simulink model "soc_WLAN_fpga"  (R2024b)
settings: Solver=FixedStepDiscrete  StartTime=0.0  StopTime=stopTime  RelTol=1e-3
PreLoadFcn:
  | addpath(fullfile(matlabroot,'toolbox','whdl','whdlexamples','whdlexamples'));
InitFcn:
  | addpath(fullfile(matlabroot,'toolbox','whdl','whdlexamples','whdlexamples'));
model workspace (MAT data in the model file):
  socvcb : containers.Map (value not decoded)
undefined symbols (not defined in the file): Add, bitRatePerOfdmSym, chanBW, coe, cpLen, dataUpsampleFactor, DelayValMaxNsdMinusLastPilotSc, DescramblerInitialSeed, designMultirateFIR, fftLen, filterLatency, filterUpsampleFactor, Fs, Hd, HT_MFMCS0, HT_MFMCS1, HT_MFMCS2, HT_MFMCS3, HT_MFMCS4, HT_MFMCS5, HT_MFMCS6, HT_MFMCS7, HTUnUsedScInd, inputSamplingRate, interp_coeff, maxPilotRefCounterVale, maxPilotsRef, maxPilotsRefNonHT, Ncol_HT, Ncol_NonHT, noDataSubCarriers, Non_HTMCS0, Non_HTMCS1, Non_HTMCS2, Non_HTMCS3, Non_HTMCS4, Non_HTMCS5, Non_HTMCS6, Non_HTMCS7, Nrow_HT, Nrow_NonHT, numDSC_HT, numDSC_HT_vhtSigB, numDSC_NonHT, numDscHT, numDscNonHT, numOfBitsPerOFDMSym, numOfDataBitsPerOFDMSym, numPilots, numScHT, numSCS_HT, numSCS_NonHT, pnSeq, QAM, rxDownsampleFactor, secondPIdx_HT, secondPIdx_NonHT, Shift, VHTMCS0, VHTMCS1 ... (+7)
libraries: hdlsllib x267, simulink x210, dspsigops x22, whdlutilities x10, whdlmod x9, dsphdlfiltering2 x5, dsphdlmathfun2 x4, whdledac x3, hwlogicconnlib x2, commhdlcrc x2, dsphdlsigops2 x2
(part 13 of 14)

== system soc_WLAN_fpga/WLAN/WLAN HDL/WLAN_Tx_Rx/WLAN_Rx/WLANHDLReceiver/DataRecovery/Deinterleaver/DeInterleaver_NonHT/Stage 2 64QAM/Read Logic/Generate Read Address/Read Address of Deinterleaver/Generate Read Address ==
  note: Compute read address
  blockLen : Inport
  enable : Inport  Port=2
  reset : Inport  Port=3
  Add : Sum
  Add1 : Sum  OutDataTypeStr=fixdt(0,nextpow2(maxBlkSize),0)
  Constant : Constant  OutDataTypeStr=fixdt(0,1,0)  SampleTime=-1
  Constant1 : Constant  Value=nColumns-2  OutDataTypeStr=Inherit: Inherit via back propagation  SampleTime=-1
  Constant2 : Constant  Value=nColumns  OutDataTypeStr=fixdt(0,nextpow2(nColumns+1),0)  SampleTime=-1
  Constant4 : Constant  Value=nColumns  OutDataTypeStr=Inherit: Inherit via back propagation  SampleTime=-1
  Delay{,4..6,10..12,14..16} (10 alike) : Delay  DelayLength=1
  Delay{1..3,13} (4 alike) : Delay
  Divide : Product  Inputs=*/  OutDataTypeStr=fixdt(0,nextpow2(maxNRows+1),0)  RndMeth=Zero  SaturateOnIntegerOverflow=on
  From : From
  Goto : Goto
  HDL Counter2 : hdlsllib/Sources/HDL Counter  CountType=Count limited  CountInit=0  CountStep=1  CountMax=maxBlkSize  CountFromType=Initial value  CountFrom=0  CountResetPort=on  CountLoadPort=off  CountEnbPort=on  CountDirPort=off  CountHitOutputPort=off  CountDataType=Unsigned  CountWordLen=nextpow2(maxBlkSize+1)  CountFracLen=0  CountSampTime=1
  Logical Operator : Logic  Operator=OR  IconShape=distinctive  AllPortsSameDT=off  OutDataTypeStr=boolean
  Logical Operator1 : Logic  IconShape=distinctive  AllPortsSameDT=off  OutDataTypeStr=boolean
  Product : Product  OutDataTypeStr=fixdt(0,nextpow2(maxBlkSize),0)
  Relational Operator : RelationalOperator  Operator===  OutDataTypeStr=boolean  InputSameDT=off
  Relational Operator1 : RelationalOperator  OutDataTypeStr=boolean  InputSameDT=off
  Switch : Switch  Criteria=u2 ~= 0  SaturateOnIntegerOverflow=off  InputSameDT=off
  colCounter : hdlsllib/Sources/HDL Counter  CountType=Count limited  CountInit=0  CountStep=1  CountMax=maxNRows -1  CountFromType=Initial value  CountFrom=0  CountResetPort=on  CountLoadPort=off  CountEnbPort=on  CountDirPort=off  CountHitOutputPort=off  CountDataType=Unsigned  CountWordLen=nextpow2(maxNRows)  CountFracLen=0  CountSampTime=1
  rowCounter : hdlsllib/Sources/HDL Counter  CountType=Count limited  CountInit=0  CountStep=1  CountMax=nColumns -1  CountFromType=Initial value  CountFrom=0  CountResetPort=on  CountLoadPort=off  CountEnbPort=on  CountDirPort=off  CountHitOutputPort=off  CountDataType=Unsigned  CountWordLen=nextpow2(nColumns+1)  CountFracLen=0  CountSampTime=1
  blockDataCount : Outport
  currentAddr : Outport  Port=2
  wires:
  Relational Operator1/1 -> Logical Operator1/1
  HDL Counter2/1 -> Goto/1, Relational Operator1/2
  reset/1 -> Delay15/1, HDL Counter2/1
  Logical Operator/1 -> rowCounter/1
  Delay/1 -> Logical Operator/1, colCounter/2
  Relational Operator/1 -> Delay/1
  Constant/1 -> Add/2
  blockLen/1 -> Relational Operator1/1, Add/1
  enable/1 -> Logical Operator1/2, HDL Counter2/2
  rowCounter/1 -> Delay1/1, Relational Operator/2  "rowIndex"
  colCounter/1 -> Delay2/1  "colIndex"
  Add1/1 -> Delay6/1
  Product/1 -> Delay5/1
  Delay2/1 -> Delay4/1
  Delay4/1 -> Add1/2
  Delay5/1 -> Add1/1
  Delay15/1 -> colCounter/1, Logical Operator/2
  Delay16/1 -> Switch/2, rowCounter/2
  Delay13/1 -> Delay14/1
  Delay14/1 -> Delay11/1
  Delay12/1 -> Delay13/1
  Delay6/1 -> currentAddr/1
  Delay11/1 -> blockDataCount/1
  Add/1 -> Delay10/1
  From/1 -> Delay12/1
  Logical Operator1/1 -> Delay16/1
  Divide/1 -> Delay3/1
  Delay10/1 -> Divide/1
  Constant2/1 -> Divide/2
  Switch/1 -> Relational Operator/1
  Constant1/1 -> Switch/1
  Constant4/1 -> Switch/3
  Delay1/1 -> Product/2
  Delay3/1 -> Product/1

== system soc_WLAN_fpga/WLAN/WLAN HDL/WLAN_Tx_Rx/WLAN_Rx/WLANHDLReceiver/DataRecovery/Deinterleaver/DeInterleaver_NonHT/Stage 2 64QAM/Read Logic/Generate Read Address/Read Address of Interleaver/Generate Read Address ==
  note: Compute read address
  blockLen : Inport
  enable : Inport  Port=2
  reset : Inport  Port=3
  Add : Sum
  Add1 : Sum  Inputs=+-  OutDataTypeStr=Inherit: Inherit via back propagation
  Add2 : Sum  OutDataTypeStr=fixdt(0,nextpow2(maxBlkSize),0)
  Constant : Constant  OutDataTypeStr=fixdt(0,1,0)  SampleTime=-1
  Constant1 : Constant  Value=2  OutDataTypeStr=fixdt(0,2,0)  SampleTime=-1
  Constant2 : Constant  Value=nColumns  OutDataTypeStr=fixdt(0,nextpow2(nColumns+1),0)  SampleTime=-1
  Constant3 : Constant  Value=nColumns  OutDataTypeStr=fixdt(0,nextpow2(nColumns+1),0)  SampleTime=-1
  Constant4 : Constant  Value=maxNRows  OutDataTypeStr=Inherit: Inherit via back propagation  SampleTime=-1
  Delay{,1..16} (17 alike) : Delay  DelayLength=1
  Divide : Product  Inputs=*/  OutDataTypeStr=fixdt(0,nextpow2(maxNRows+1),0)  RndMeth=Zero  SaturateOnIntegerOverflow=on
  From : From
  Goto : Goto
  HDL Counter2 : hdlsllib/Sources/HDL Counter  CountType=Count limited  CountInit=0  CountStep=1  CountMax=maxBlkSize  CountFromType=Initial value  CountFrom=0  CountResetPort=on  CountLoadPort=off  CountEnbPort=on  CountDirPort=off  CountHitOutputPort=off  CountDataType=Unsigned  CountWordLen=nextpow2(maxBlkSize+1)  CountFracLen=0  CountSampTime=1
  Logical Operator : Logic  Operator=OR  IconShape=distinctive  AllPortsSameDT=off  OutDataTypeStr=boolean
  Logical Operator1 : Logic  IconShape=distinctive  AllPortsSameDT=off  OutDataTypeStr=boolean
  Product : Product  OutDataTypeStr=fixdt(0,nextpow2(maxBlkSize),0)
  Relational Operator : RelationalOperator  Operator===  OutDataTypeStr=boolean  InputSameDT=off
  Relational Operator1 : RelationalOperator  OutDataTypeStr=boolean  InputSameDT=off
  Switch : Switch  Criteria=u2 ~= 0  SaturateOnIntegerOverflow=off  InputSameDT=off
  colCounter : hdlsllib/Sources/HDL Counter  CountType=Count limited  CountInit=0  CountStep=1  CountMax=nColumns -1  CountFromType=Initial value  CountFrom=0  CountResetPort=on  CountLoadPort=off  CountEnbPort=on  CountDirPort=off  CountHitOutputPort=off  CountDataType=Unsigned  CountWordLen=nextpow2(nColumns)  CountFracLen=0  CountSampTime=1
  rowCounter : hdlsllib/Sources/HDL Counter  CountType=Count limited  CountInit=0  CountStep=1  CountMax=maxNRows -1  CountFromType=Initial value  CountFrom=0  CountResetPort=on  CountLoadPort=off  CountEnbPort=on  CountDirPort=off  CountHitOutputPort=off  CountDataType=Unsigned  CountWordLen=nextpow2(maxNRows+1)  CountFracLen=0  CountSampTime=1
  blockDataCount : Outport
  currentAddr : Outport  Port=2
  wires:
  Constant3/1 -> Product/2
  Delay9/1 -> Delay13/1
  Delay8/1 -> rowCounter/2, Switch/2
  Delay7/1 -> Logical Operator/2, colCounter/1
  Delay3/1 -> Add1/1
  Delay1/1 -> Product/1
  Add1/1 -> Switch/1
  Constant1/1 -> Add1/2
  Divide/1 -> Delay3/1
  Constant4/1 -> Switch/3
  Switch/1 -> Relational Operator/1
  Constant2/1 -> Divide/2
  Delay10/1 -> Divide/1
  Logical Operator1/1 -> Delay16/1
  From/1 -> Delay12/1
  Add/1 -> Delay10/1
  Delay11/1 -> blockDataCount/1
  Delay6/1 -> currentAddr/1
  Delay12/1 -> Delay9/1
  Delay14/1 -> Delay11/1
  Delay13/1 -> Delay14/1
  Delay16/1 -> Delay8/1
  Delay15/1 -> Delay7/1
  Delay5/1 -> Add2/1
  Delay4/1 -> Add2/2
  Delay2/1 -> Delay4/1
  Product/1 -> Delay5/1
  Add2/1 -> Delay6/1
  colCounter/1 -> Delay2/1  "colIndex"
  rowCounter/1 -> Delay1/1, Relational Operator/2  "rowIndex"
  enable/1 -> HDL Counter2/2, Logical Operator1/2
  blockLen/1 -> Add/1, Relational Operator1/1
  Constant/1 -> Add/2
  Relational Operator/1 -> Delay/1
  Delay/1 -> colCounter/2, Logical Operator/1
  Logical Operator/1 -> rowCounter/1
  reset/1 -> HDL Counter2/1, Delay15/1
  HDL Counter2/1 -> Relational Operator1/2, Goto/1
  Relational Operator1/1 -> Logical Operator1/1

== system soc_WLAN_fpga/WLAN/WLAN HDL/WLAN_Tx_Rx/WLAN_Rx/WLANHDLReceiver/DataRecovery/Deinterleaver/DeInterleaver_NonHT/Stage 2 BPSK/Read Logic/Generate Read Address/Read Address of Deinterleaver/Generate Read Address ==
  note: Compute read address
  blockLen : Inport
  enable : Inport  Port=2
  reset : Inport  Port=3
  Add : Sum
  Add1 : Sum  OutDataTypeStr=fixdt(0,nextpow2(maxBlkSize),0)
  Constant : Constant  OutDataTypeStr=fixdt(0,1,0)  SampleTime=-1
  Constant1 : Constant  Value=nColumns-2  OutDataTypeStr=Inherit: Inherit via back propagation  SampleTime=-1
  Constant2 : Constant  Value=nColumns  OutDataTypeStr=fixdt(0,nextpow2(nColumns+1),0)  SampleTime=-1
  Constant4 : Constant  Value=nColumns  OutDataTypeStr=Inherit: Inherit via back propagation  SampleTime=-1
  Delay{,4..6,10..12,14..16} (10 alike) : Delay  DelayLength=1
  Delay{1..3,13} (4 alike) : Delay
  Divide : Product  Inputs=*/  OutDataTypeStr=fixdt(0,nextpow2(maxNRows+1),0)  RndMeth=Zero  SaturateOnIntegerOverflow=on
  From : From
  Goto : Goto
  HDL Counter2 : hdlsllib/Sources/HDL Counter  CountType=Count limited  CountInit=0  CountStep=1  CountMax=maxBlkSize  CountFromType=Initial value  CountFrom=0  CountResetPort=on  CountLoadPort=off  CountEnbPort=on  CountDirPort=off  CountHitOutputPort=off  CountDataType=Unsigned  CountWordLen=nextpow2(maxBlkSize+1)  CountFracLen=0  CountSampTime=1
  Logical Operator : Logic  Operator=OR  IconShape=distinctive  AllPortsSameDT=off  OutDataTypeStr=boolean
  Logical Operator1 : Logic  IconShape=distinctive  AllPortsSameDT=off  OutDataTypeStr=boolean
  Product : Product  OutDataTypeStr=fixdt(0,nextpow2(maxBlkSize),0)
  Relational Operator : RelationalOperator  Operator===  OutDataTypeStr=boolean  InputSameDT=off
  Relational Operator1 : RelationalOperator  OutDataTypeStr=boolean  InputSameDT=off
  Switch : Switch  Criteria=u2 ~= 0  SaturateOnIntegerOverflow=off  InputSameDT=off
  colCounter : hdlsllib/Sources/HDL Counter  CountType=Count limited  CountInit=0  CountStep=1  CountMax=maxNRows -1  CountFromType=Initial value  CountFrom=0  CountResetPort=on  CountLoadPort=off  CountEnbPort=on  CountDirPort=off  CountHitOutputPort=off  CountDataType=Unsigned  CountWordLen=nextpow2(maxNRows)  CountFracLen=0  CountSampTime=1
  rowCounter : hdlsllib/Sources/HDL Counter  CountType=Count limited  CountInit=0  CountStep=1  CountMax=nColumns -1  CountFromType=Initial value  CountFrom=0  CountResetPort=on  CountLoadPort=off  CountEnbPort=on  CountDirPort=off  CountHitOutputPort=off  CountDataType=Unsigned  CountWordLen=nextpow2(nColumns+1)  CountFracLen=0  CountSampTime=1
  blockDataCount : Outport
  currentAddr : Outport  Port=2
  wires:
  Relational Operator1/1 -> Logical Operator1/1
  HDL Counter2/1 -> Goto/1, Relational Operator1/2
  reset/1 -> Delay15/1, HDL Counter2/1
  Logical Operator/1 -> rowCounter/1
  Delay/1 -> Logical Operator/1, colCounter/2
  Relational Operator/1 -> Delay/1
  Constant/1 -> Add/2
  blockLen/1 -> Relational Operator1/1, Add/1
  enable/1 -> Logical Operator1/2, HDL Counter2/2
  rowCounter/1 -> Delay1/1, Relational Operator/2  "rowIndex"
  colCounter/1 -> Delay2/1  "colIndex"
  Add1/1 -> Delay6/1
  Product/1 -> Delay5/1
  Delay2/1 -> Delay4/1
  Delay4/1 -> Add1/2
  Delay5/1 -> Add1/1
  Delay15/1 -> colCounter/1, Logical Operator/2
  Delay16/1 -> Switch/2, rowCounter/2
  Delay13/1 -> Delay14/1
  Delay14/1 -> Delay11/1
  Delay12/1 -> Delay13/1
  Delay6/1 -> currentAddr/1
  Delay11/1 -> blockDataCount/1
  Add/1 -> Delay10/1
  From/1 -> Delay12/1
  Logical Operator1/1 -> Delay16/1
  Divide/1 -> Delay3/1
  Delay10/1 -> Divide/1
  Constant2/1 -> Divide/2
  Switch/1 -> Relational Operator/1
  Constant1/1 -> Switch/1
  Constant4/1 -> Switch/3
  Delay1/1 -> Product/2
  Delay3/1 -> Product/1

== system soc_WLAN_fpga/WLAN/WLAN HDL/WLAN_Tx_Rx/WLAN_Rx/WLANHDLReceiver/DataRecovery/Deinterleaver/DeInterleaver_NonHT/Stage 2 BPSK/Read Logic/Generate Read Address/Read Address of Interleaver/Generate Read Address ==
  note: Compute read address
  blockLen : Inport
  enable : Inport  Port=2
  reset : Inport  Port=3
  Add : Sum
  Add1 : Sum  Inputs=+-  OutDataTypeStr=Inherit: Inherit via back propagation
  Add2 : Sum  OutDataTypeStr=fixdt(0,nextpow2(maxBlkSize),0)
  Constant : Constant  OutDataTypeStr=fixdt(0,1,0)  SampleTime=-1
  Constant1 : Constant  Value=2  OutDataTypeStr=fixdt(0,2,0)  SampleTime=-1
  Constant2 : Constant  Value=nColumns  OutDataTypeStr=fixdt(0,nextpow2(nColumns+1),0)  SampleTime=-1
  Constant3 : Constant  Value=nColumns  OutDataTypeStr=fixdt(0,nextpow2(nColumns+1),0)  SampleTime=-1
  Constant4 : Constant  Value=maxNRows  OutDataTypeStr=Inherit: Inherit via back propagation  SampleTime=-1
  Delay{,1..16} (17 alike) : Delay  DelayLength=1
  Divide : Product  Inputs=*/  OutDataTypeStr=fixdt(0,nextpow2(maxNRows+1),0)  RndMeth=Zero  SaturateOnIntegerOverflow=on
  From : From
  Goto : Goto
  HDL Counter2 : hdlsllib/Sources/HDL Counter  CountType=Count limited  CountInit=0  CountStep=1  CountMax=maxBlkSize  CountFromType=Initial value  CountFrom=0  CountResetPort=on  CountLoadPort=off  CountEnbPort=on  CountDirPort=off  CountHitOutputPort=off  CountDataType=Unsigned  CountWordLen=nextpow2(maxBlkSize+1)  CountFracLen=0  CountSampTime=1
  Logical Operator : Logic  Operator=OR  IconShape=distinctive  AllPortsSameDT=off  OutDataTypeStr=boolean
  Logical Operator1 : Logic  IconShape=distinctive  AllPortsSameDT=off  OutDataTypeStr=boolean
  Product : Product  OutDataTypeStr=fixdt(0,nextpow2(maxBlkSize),0)
  Relational Operator : RelationalOperator  Operator===  OutDataTypeStr=boolean  InputSameDT=off
  Relational Operator1 : RelationalOperator  OutDataTypeStr=boolean  InputSameDT=off
  Switch : Switch  Criteria=u2 ~= 0  SaturateOnIntegerOverflow=off  InputSameDT=off
  colCounter : hdlsllib/Sources/HDL Counter  CountType=Count limited  CountInit=0  CountStep=1  CountMax=nColumns -1  CountFromType=Initial value  CountFrom=0  CountResetPort=on  CountLoadPort=off  CountEnbPort=on  CountDirPort=off  CountHitOutputPort=off  CountDataType=Unsigned  CountWordLen=nextpow2(nColumns)  CountFracLen=0  CountSampTime=1
  rowCounter : hdlsllib/Sources/HDL Counter  CountType=Count limited  CountInit=0  CountStep=1  CountMax=maxNRows -1  CountFromType=Initial value  CountFrom=0  CountResetPort=on  CountLoadPort=off  CountEnbPort=on  CountDirPort=off  CountHitOutputPort=off  CountDataType=Unsigned  CountWordLen=nextpow2(maxNRows+1)  CountFracLen=0  CountSampTime=1
  blockDataCount : Outport
  currentAddr : Outport  Port=2
  wires:
  Constant3/1 -> Product/2
  Delay9/1 -> Delay13/1
  Delay8/1 -> rowCounter/2, Switch/2
  Delay7/1 -> Logical Operator/2, colCounter/1
  Delay3/1 -> Add1/1
  Delay1/1 -> Product/1
  Add1/1 -> Switch/1
  Constant1/1 -> Add1/2
  Divide/1 -> Delay3/1
  Constant4/1 -> Switch/3
  Switch/1 -> Relational Operator/1
  Constant2/1 -> Divide/2
  Delay10/1 -> Divide/1
  Logical Operator1/1 -> Delay16/1
  From/1 -> Delay12/1
  Add/1 -> Delay10/1
  Delay11/1 -> blockDataCount/1
  Delay6/1 -> currentAddr/1
  Delay12/1 -> Delay9/1
  Delay14/1 -> Delay11/1
  Delay13/1 -> Delay14/1
  Delay16/1 -> Delay8/1
  Delay15/1 -> Delay7/1
  Delay5/1 -> Add2/1
  Delay4/1 -> Add2/2
  Delay2/1 -> Delay4/1
  Product/1 -> Delay5/1
  Add2/1 -> Delay6/1
  colCounter/1 -> Delay2/1  "colIndex"
  rowCounter/1 -> Delay1/1, Relational Operator/2  "rowIndex"
  enable/1 -> HDL Counter2/2, Logical Operator1/2
  blockLen/1 -> Add/1, Relational Operator1/1
  Constant/1 -> Add/2
  Relational Operator/1 -> Delay/1
  Delay/1 -> colCounter/2, Logical Operator/1
  Logical Operator/1 -> rowCounter/1
  reset/1 -> HDL Counter2/1, Delay15/1
  HDL Counter2/1 -> Relational Operator1/2, Goto/1
  Relational Operator1/1 -> Logical Operator1/1

== system soc_WLAN_fpga/WLAN/WLAN HDL/WLAN_Tx_Rx/WLAN_Rx/WLANHDLReceiver/DataRecovery/Deinterleaver/DeInterleaver_NonHT/Stage 2 QPSK/Read Logic/Generate Read Address/Read Address of Deinterleaver/Generate Read Address ==
  note: Compute read address
  blockLen : Inport
  enable : Inport  Port=2
  reset : Inport  Port=3
  Add : Sum
  Add1 : Sum  OutDataTypeStr=fixdt(0,nextpow2(maxBlkSize),0)
  Constant : Constant  OutDataTypeStr=fixdt(0,1,0)  SampleTime=-1
  Constant1 : Constant  Value=nColumns-2  OutDataTypeStr=Inherit: Inherit via back propagation  SampleTime=-1
  Constant2 : Constant  Value=nColumns  OutDataTypeStr=fixdt(0,nextpow2(nColumns+1),0)  SampleTime=-1
  Constant4 : Constant  Value=nColumns  OutDataTypeStr=Inherit: Inherit via back propagation  SampleTime=-1
  Delay{,4..6,10..12,14..16} (10 alike) : Delay  DelayLength=1
  Delay{1..3,13} (4 alike) : Delay
  Divide : Product  Inputs=*/  OutDataTypeStr=fixdt(0,nextpow2(maxNRows+1),0)  RndMeth=Zero  SaturateOnIntegerOverflow=on
  From : From
  Goto : Goto
  HDL Counter2 : hdlsllib/Sources/HDL Counter  CountType=Count limited  CountInit=0  CountStep=1  CountMax=maxBlkSize  CountFromType=Initial value  CountFrom=0  CountResetPort=on  CountLoadPort=off  CountEnbPort=on  CountDirPort=off  CountHitOutputPort=off  CountDataType=Unsigned  CountWordLen=nextpow2(maxBlkSize+1)  CountFracLen=0  CountSampTime=1
  Logical Operator : Logic  Operator=OR  IconShape=distinctive  AllPortsSameDT=off  OutDataTypeStr=boolean
  Logical Operator1 : Logic  IconShape=distinctive  AllPortsSameDT=off  OutDataTypeStr=boolean
  Product : Product  OutDataTypeStr=fixdt(0,nextpow2(maxBlkSize),0)
  Relational Operator : RelationalOperator  Operator===  OutDataTypeStr=boolean  InputSameDT=off
  Relational Operator1 : RelationalOperator  OutDataTypeStr=boolean  InputSameDT=off
  Switch : Switch  Criteria=u2 ~= 0  SaturateOnIntegerOverflow=off  InputSameDT=off
  colCounter : hdlsllib/Sources/HDL Counter  CountType=Count limited  CountInit=0  CountStep=1  CountMax=maxNRows -1  CountFromType=Initial value  CountFrom=0  CountResetPort=on  CountLoadPort=off  CountEnbPort=on  CountDirPort=off  CountHitOutputPort=off  CountDataType=Unsigned  CountWordLen=nextpow2(maxNRows)  CountFracLen=0  CountSampTime=1
  rowCounter : hdlsllib/Sources/HDL Counter  CountType=Count limited  CountInit=0  CountStep=1  CountMax=nColumns -1  CountFromType=Initial value  CountFrom=0  CountResetPort=on  CountLoadPort=off  CountEnbPort=on  CountDirPort=off  CountHitOutputPort=off  CountDataType=Unsigned  CountWordLen=nextpow2(nColumns+1)  CountFracLen=0  CountSampTime=1
  blockDataCount : Outport
  currentAddr : Outport  Port=2
  wires:
  Relational Operator1/1 -> Logical Operator1/1
  HDL Counter2/1 -> Goto/1, Relational Operator1/2
  reset/1 -> Delay15/1, HDL Counter2/1
  Logical Operator/1 -> rowCounter/1
  Delay/1 -> Logical Operator/1, colCounter/2
  Relational Operator/1 -> Delay/1
  Constant/1 -> Add/2
  blockLen/1 -> Relational Operator1/1, Add/1
  enable/1 -> Logical Operator1/2, HDL Counter2/2
  rowCounter/1 -> Delay1/1, Relational Operator/2  "rowIndex"
  colCounter/1 -> Delay2/1  "colIndex"
  Add1/1 -> Delay6/1
  Product/1 -> Delay5/1
  Delay2/1 -> Delay4/1
  Delay4/1 -> Add1/2
  Delay5/1 -> Add1/1
  Delay15/1 -> colCounter/1, Logical Operator/2
  Delay16/1 -> Switch/2, rowCounter/2
  Delay13/1 -> Delay14/1
  Delay14/1 -> Delay11/1
  Delay12/1 -> Delay13/1
  Delay6/1 -> currentAddr/1
  Delay11/1 -> blockDataCount/1
  Add/1 -> Delay10/1
  From/1 -> Delay12/1
  Logical Operator1/1 -> Delay16/1
  Divide/1 -> Delay3/1
  Delay10/1 -> Divide/1
  Constant2/1 -> Divide/2
  Switch/1 -> Relational Operator/1
  Constant1/1 -> Switch/1
  Constant4/1 -> Switch/3
  Delay1/1 -> Product/2
  Delay3/1 -> Product/1

== system soc_WLAN_fpga/WLAN/WLAN HDL/WLAN_Tx_Rx/WLAN_Rx/WLANHDLReceiver/DataRecovery/Deinterleaver/DeInterleaver_NonHT/Stage 2 QPSK/Read Logic/Generate Read Address/Read Address of Interleaver/Generate Read Address ==
  note: Compute read address
  blockLen : Inport
  enable : Inport  Port=2
  reset : Inport  Port=3
  Add : Sum
  Add1 : Sum  Inputs=+-  OutDataTypeStr=Inherit: Inherit via back propagation
  Add2 : Sum  OutDataTypeStr=fixdt(0,nextpow2(maxBlkSize),0)
  Constant : Constant  OutDataTypeStr=fixdt(0,1,0)  SampleTime=-1
  Constant1 : Constant  Value=2  OutDataTypeStr=fixdt(0,2,0)  SampleTime=-1
  Constant2 : Constant  Value=nColumns  OutDataTypeStr=fixdt(0,nextpow2(nColumns+1),0)  SampleTime=-1
  Constant3 : Constant  Value=nColumns  OutDataTypeStr=fixdt(0,nextpow2(nColumns+1),0)  SampleTime=-1
  Constant4 : Constant  Value=maxNRows  OutDataTypeStr=Inherit: Inherit via back propagation  SampleTime=-1
  Delay{,1..16} (17 alike) : Delay  DelayLength=1
  Divide : Product  Inputs=*/  OutDataTypeStr=fixdt(0,nextpow2(maxNRows+1),0)  RndMeth=Zero  SaturateOnIntegerOverflow=on
  From : From
  Goto : Goto
  HDL Counter2 : hdlsllib/Sources/HDL Counter  CountType=Count limited  CountInit=0  CountStep=1  CountMax=maxBlkSize  CountFromType=Initial value  CountFrom=0  CountResetPort=on  CountLoadPort=off  CountEnbPort=on  CountDirPort=off  CountHitOutputPort=off  CountDataType=Unsigned  CountWordLen=nextpow2(maxBlkSize+1)  CountFracLen=0  CountSampTime=1
  Logical Operator : Logic  Operator=OR  IconShape=distinctive  AllPortsSameDT=off  OutDataTypeStr=boolean
  Logical Operator1 : Logic  IconShape=distinctive  AllPortsSameDT=off  OutDataTypeStr=boolean
  Product : Product  OutDataTypeStr=fixdt(0,nextpow2(maxBlkSize),0)
  Relational Operator : RelationalOperator  Operator===  OutDataTypeStr=boolean  InputSameDT=off
  Relational Operator1 : RelationalOperator  OutDataTypeStr=boolean  InputSameDT=off
  Switch : Switch  Criteria=u2 ~= 0  SaturateOnIntegerOverflow=off  InputSameDT=off
  colCounter : hdlsllib/Sources/HDL Counter  CountType=Count limited  CountInit=0  CountStep=1  CountMax=nColumns -1  CountFromType=Initial value  CountFrom=0  CountResetPort=on  CountLoadPort=off  CountEnbPort=on  CountDirPort=off  CountHitOutputPort=off  CountDataType=Unsigned  CountWordLen=nextpow2(nColumns)  CountFracLen=0  CountSampTime=1
  rowCounter : hdlsllib/Sources/HDL Counter  CountType=Count limited  CountInit=0  CountStep=1  CountMax=maxNRows -1  CountFromType=Initial value  CountFrom=0  CountResetPort=on  CountLoadPort=off  CountEnbPort=on  CountDirPort=off  CountHitOutputPort=off  CountDataType=Unsigned  CountWordLen=nextpow2(maxNRows+1)  CountFracLen=0  CountSampTime=1
  blockDataCount : Outport
  currentAddr : Outport  Port=2
  wires:
  Constant3/1 -> Product/2
  Delay9/1 -> Delay13/1
  Delay8/1 -> rowCounter/2, Switch/2
  Delay7/1 -> Logical Operator/2, colCounter/1
  Delay3/1 -> Add1/1
  Delay1/1 -> Product/1
  Add1/1 -> Switch/1
  Constant1/1 -> Add1/2
  Divide/1 -> Delay3/1
  Constant4/1 -> Switch/3
  Switch/1 -> Relational Operator/1
  Constant2/1 -> Divide/2
  Delay10/1 -> Divide/1
  Logical Operator1/1 -> Delay16/1
  From/1 -> Delay12/1
  Add/1 -> Delay10/1
  Delay11/1 -> blockDataCount/1
  Delay6/1 -> currentAddr/1
  Delay12/1 -> Delay9/1
  Delay14/1 -> Delay11/1
  Delay13/1 -> Delay14/1
  Delay16/1 -> Delay8/1
  Delay15/1 -> Delay7/1
  Delay5/1 -> Add2/1
  Delay4/1 -> Add2/2
  Delay2/1 -> Delay4/1
  Product/1 -> Delay5/1
  Add2/1 -> Delay6/1
  colCounter/1 -> Delay2/1  "colIndex"
  rowCounter/1 -> Delay1/1, Relational Operator/2  "rowIndex"
  enable/1 -> HDL Counter2/2, Logical Operator1/2
  blockLen/1 -> Add/1, Relational Operator1/1
  Constant/1 -> Add/2
  Relational Operator/1 -> Delay/1
  Delay/1 -> colCounter/2, Logical Operator/1
  Logical Operator/1 -> rowCounter/1
  reset/1 -> HDL Counter2/1, Delay15/1
  HDL Counter2/1 -> Relational Operator1/2, Goto/1
  Relational Operator1/1 -> Logical Operator1/1

== matlab function soc_WLAN_fpga/WLAN/WLAN HDL/WLAN_Tx_Rx/WLAN_Rx/WLANHDLReceiver/OFDMDemodulation/OFDMDemodParamsCalculator ==
  data: valid input; fftLen output; cpLen output; lgSc output; rgSc output; reset input; chanBW parameter
function [fftLen,cpLen,lgSc,rgSc] = OFDMDemodParamsCalculator(valid,reset,chanBW)
%#codegen

persistent countVal;
persistent count;

if isempty(count)
    count = uint16(0);
end
if valid
    count(:) = count+1;
end
if isempty(countVal)
    countVal = uint16(0);
end
if reset
    countVal = uint16(0);
end
if valid
    countVal(:) = countVal+1;
end
if chanBW==1
    if countVal > 2*80 && countVal <= 2*80+(64+32) % L-LTF1 samples
        cpLen = fi(32,0,7,0);
    elseif countVal > 2*80+(64+32) && countVal <= 4*80 % L-LTF2 samples
        cpLen = fi(0,0,7,0);
    else
        cpLen = fi(16,0,7,0); % From L-Sig Duration
    end
    % Choosing HT/VHT subcarriers to support all three frame formats
    fftLen = fi(64,0,8,0);
    lgSc = fi(0,0,3,0);
    rgSc = fi(0,0,3,0);
else % strcmp(chanBW,'40MHz') % 40MHz
    ofdmLen = 160;
    if countVal >= 2*ofdmLen && countVal < 2*ofdmLen+(128+64) % L-LTF1 samples
        cpLen = fi(64,0,7,0);
    elseif countVal >= 2*ofdmLen+(128+64) && countVal < 4*ofdmLen % L-LTF2 samples
        cpLen = fi(0,0,7,0);
    else
        cpLen = fi(32,0,7,0); % From L-Sig Duration
    end
    % Choosing HT/VHT subcarriers to support all three frame formats
    fftLen = fi(128,0,8,0);
    lgSc = fi(0,0,3,0);
    rgSc = fi(0,0,3,0);
    
end
end

== matlab function soc_WLAN_fpga/WLAN/WLAN HDL/WLAN_Tx_Rx/WLAN_Rx/WLANHDLReceiver/WLANTimeAndFrequencySynchronization/Coarse Time Sync/correlator/delayedCorrelation/DTadjust ==
  data: in input; out output; wlanConfig parameter
function out = DTadjust(in,wlanConfig)
%#codegen
if isfloat(in)
    out = in;
else
    WL = in.WordLength;
    FL = WL - (log2(wlanConfig.lstfLen)+1)-1;
    out = fi(in,1,WL,FL);
end

== matlab function soc_WLAN_fpga/WLAN/WLAN HDL/WLAN_Tx_Rx/WLAN_Rx/WLANHDLReceiver/WLANTimeAndFrequencySynchronization/Coarse Time Sync/energyCalculator/magnitudeSquared/MagnitudeSquared/DTadjust ==
  data: in input; out output; wlanConfig parameter
function out = DTadjust(in,wlanConfig)
%#codegen
if isfloat(in)
    out = in;
else
    WL = in.WordLength;
    FL = WL - (log2(wlanConfig.lstfLen)+1)-1;
    out = fi(in,1,WL,FL);
end

== matlab function soc_WLAN_fpga/WLAN/WLAN HDL/WLAN_Tx_Rx/WLAN_Rx/WLANHDLReceiver/NonHTCPEEstAndCorrection/CPEEstimator/sampleAndHold ==
  data: x input; y output; enb input; rst input
function y = sampleAndHold(x,enb,rst)
%#codegen

persistent xReg;
if isempty(xReg) || rst
    xReg = cast(0,'like',x);
end

if enb == 1
    xReg = x;
    y = x;
else
    y = xReg;
end

== matlab function soc_WLAN_fpga/WLAN/WLAN HDL/WLAN_Tx_Rx/WLAN_Rx/WLANHDLReceiver/WLANTimeAndFrequencySynchronization/Fine Time Sync/peakSearcher/maxPeakSearcher/maxPeakSearcher ==
  data: dataIn input; maxPeak output; validIn input; countValue input; reset input; wlanConfig parameter
function maxPeak  = maxPeakSearcher(dataIn,validIn,countValue,reset,wlanConfig)
%#codegen

persistent maxPeakReg;
persistent maxPeakPrev;
persistent maxValueReg;

if isempty(maxPeakReg) || reset
    maxValueReg = cast(0,'like',dataIn);
    maxPeakReg = cast(0,'like',countValue);
    maxPeakPrev = cast(0,'like',countValue);
end

if validIn
    if dataIn > maxValueReg        
       maxPeakReg = countValue;
       maxValueReg = dataIn;
    end
end

if countValue == 2*wlanConfig.corrLen-1
    maxPeak  = maxPeakReg-wlanConfig.corrLen;
    maxPeakPrev = maxPeak;
else
    maxPeak  = cast(maxPeakPrev,'like',countValue);
end

== matlab function soc_WLAN_fpga/WLAN/WLAN HDL/WLAN_Tx_Rx/WLAN_Rx/WLANHDLReceiver/WLANTimeAndFrequencySynchronization/Fine Time Sync/peakSearcher/peakDetector/dataSelector  ==
  data: syncEn input; dataIn input; dataOut output; validIn input
function dataOut = dataSelector(syncEn,dataIn,validIn)
%#codegen

if validIn && syncEn
    dataOut = dataIn;
else
    dataOut = cast(complex(0,0),'like',dataIn);
end

== matlab function soc_WLAN_fpga/WLAN/WLAN HDL/WLAN_Tx_Rx/WLAN_Rx/WLANHDLReceiver/WLANTimeAndFrequencySynchronization/Coarse Time Sync/peakDetection/MATLAB Function1 ==
  data: syncEn input; dataIn input; dataOut output; validIn input
function dataOut = dataSelector(syncEn,dataIn,validIn)
%#codegen

if validIn && syncEn
    dataOut = dataIn;
else
    dataOut = cast(complex(0,0),'like',dataIn);
end

== matlab function soc_WLAN_fpga/WLAN/WLAN HDL/WLAN_Tx_Rx/WLAN_Rx/WLANHDLReceiver/WLANTimeAndFrequencySynchronization/Coarse Time Sync/peakDetection/searchStartOfFrame ==
  data: thresholdValid input; valid input; syncOut output; wlanConfig parameter
function syncOut  = searchStartOfFrame(thresholdValid,valid,wlanConfig)
%#codegen
persistent countVal;
persistent countEnb;
persistent validCount;
persistent detectFlag;
persistent detectFlagCount;

WL = ceil(log2(wlanConfig.lstfLen*10));
if isempty(countVal)
    countVal = fi(0,0,WL,0);
    countEnb = false;
end
if isempty(detectFlag)
    detectFlag = false;
    detectFlagCount = fi(0,0,WL,0);
end
if isempty(validCount)
    validCount = fi(0,0,WL,0); % Considering max count of 10 for STFs
end
if valid && thresholdValid 
    validCount(:) = validCount + 1;
    if validCount == 1
        countVal(:) = 0;
        countEnb = true;
    end
    
end
if detectFlagCount > 0
    detectFlagCount(:) = detectFlagCount+1;
end
if countEnb
    countVal(:) = countVal + 1;
    if countVal == wlanConfig.lstfLen*10+1
        countVal(:) = 0;
        countEnb = false;
        if validCount > wlanConfig.lstfLen*5
            detectFlag = true;
            detectFlagCount(:) =1;
        else
            detectFlag = false;
        end
        validCount(:) = 0;
    end
end

if detectFlagCount > wlanConfig.lstfLen*10
    detectFlagCount(:)=0;
    detectFlag = false;
end
syncOut = detectFlag;

== matlab function soc_WLAN_fpga/WLAN/WLAN HDL/WLAN_Tx_Rx/WLAN_Rx/WLANHDLReceiver/WLANTimeAndFrequencySynchronization/Coarse CFO Estimation and Correction/Coarse CFO Correction/DTConverter ==
  data: dataIn1 input; dataOut output; dataIn2 input
function dataOut = DTConverter(dataIn1,dataIn2)
%#codegen
dataOut = cast(dataIn2,'like',dataIn1);
end

== matlab function soc_WLAN_fpga/WLAN/WLAN HDL/WLAN_Tx_Rx/WLAN_Rx/WLANHDLReceiver/DataRecovery/Decoder/Depuncturer/Depuncturer1/sampleParallel1 ==
  data: dataIn input; startIn input; endIn input; dataOut output; validIn input; validOut output; reset input; enb output
function [ dataOut,validOut,enb] = sampleParallel(dataIn,startIn,endIn,validIn,reset)
%#codegen
persistent dataBuff;
persistent vecCount;
persistent searchStart;
persistent sigEnb;

if isempty(dataBuff) || reset
    dataBuff = cast(zeros(2,1),'like',dataIn);
    vecCount = uint8(0);
end
if isempty(searchStart)
    searchStart = false;
    sigEnb = false;
end
if reset
    searchStart = true;
end

if startIn && searchStart
    sigEnb = true;
end

enb = sigEnb;

if endIn && searchStart
    sigEnb = false;
end

if validIn
    vecCount(:) = vecCount + 1;
    dataBuff(vecCount) = dataIn;
end

if vecCount == 2
    dataOut = dataBuff;
    validOut = true;
    vecCount(:) = 0;
else
    dataOut = cast(zeros(2,1),'like',dataIn);
    validOut = false;
end

== matlab function soc_WLAN_fpga/WLAN/WLAN HDL/WLAN_Tx_Rx/WLAN_Rx/WLANHDLReceiver/HT_VHTCPEEstAndCorrection/CPEEstimator/sampleAndHold ==
  data: x input; y output; enb input; rst input
function y = sampleAndHold(x,enb,rst)
%#codegen

persistent xReg;
if isempty(xReg) || rst
    xReg = cast(0,'like',x);
end

if enb == 1
    xReg = x;
    y = x;
else
    y = xReg;
end

== matlab function soc_WLAN_fpga/WLAN/WLAN HDL/WLAN_Tx_Rx/WLAN_Rx/WLANHDLReceiver/DataRecovery/Deinterleaver/DeInterleaver_NonHT/Stage 2 16QAM /Generate Ready/MATLAB Function1 ==
  data: trigger input; out output; nClocks parameter
function out = holdPulse(trigger,nClocks)
%#codegen

 persistent count state;
 if isempty(count)
     count = fi(0,0,nextpow2(nClocks+2),0,hdlfimath);
     state = false;
 end
 
 
 %% Executes in current clock cycle
 if trigger
     state = true;
     count(:) = 0;
 end
 
 if(state && ~trigger)
     count(:) = count +1;
 end
 
 if(count(:) == (nClocks))
    state = false;
 end
     
 out = state;
 
end

== matlab function soc_WLAN_fpga/WLAN/WLAN HDL/WLAN_Tx_Rx/WLAN_Rx/WLANHDLReceiver/DataRecovery/Deinterleaver/DeInterleaver_NonHT/Stage 2 16QAM /Read Logic/MATLAB Function ==
  data: trigger input; out output; nClocks parameter
function out = holdPulse(trigger,nClocks)
%#codegen

 persistent count state;
 if isempty(count)
     count = fi(0,0,nextpow2(nClocks+1),0,hdlfimath);
     state = false;
 end
 
 %% Executes in next clock cycle
 if(count(:) == (nClocks))
    state = false;
 end
     
 out = state;
 
 
 %% Executes in current clock cycle
 if trigger
     state = true;
     count(:) = 0;
 end
 
 if(state && ~trigger)
     count(:) = count +1;
 end
 
end

== matlab function soc_WLAN_fpga/WLAN/WLAN HDL/WLAN_Tx_Rx/WLAN_Rx/WLANHDLReceiver/DataRecovery/Deinterleaver/DeInterleaver_NonHT/Stage 2 64QAM/Generate Ready/MATLAB Function1 ==
  data: trigger input; out output; nClocks parameter
function out = holdPulse(trigger,nClocks)
%#codegen

 persistent count state;
 if isempty(count)
     count = fi(0,0,nextpow2(nClocks+2),0,hdlfimath);
     state = false;
 end
 
 
 %% Executes in current clock cycle
 if trigger
     state = true;
     count(:) = 0;
 end
 
 if(state && ~trigger)
     count(:) = count +1;
 end
 
 if(count(:) == (nClocks))
    state = false;
 end
     
 out = state;
 
end

== matlab function soc_WLAN_fpga/WLAN/WLAN HDL/WLAN_Tx_Rx/WLAN_Rx/WLANHDLReceiver/DataRecovery/Deinterleaver/DeInterleaver_NonHT/Stage 2 64QAM/Read Logic/MATLAB Function ==
  data: trigger input; out output; nClocks parameter
function out = holdPulse(trigger,nClocks)
%#codegen

 persistent count state;
 if isempty(count)
     count = fi(0,0,nextpow2(nClocks+1),0,hdlfimath);
     state = false;
 end
 
 %% Executes in next clock cycle
 if(count(:) == (nClocks))
    state = false;
 end
     
 out = state;
 
 
 %% Executes in current clock cycle
 if trigger
     state = true;
     count(:) = 0;
 end
 
 if(state && ~trigger)
     count(:) = count +1;
 end
 
end

== matlab function soc_WLAN_fpga/WLAN/WLAN HDL/WLAN_Tx_Rx/WLAN_Rx/WLANHDLReceiver/FrameFormatDetectionAndSignalRecovery/CRCCheckAndBitInterpretation/HTSigBitRecover ==
  data: bit input; validIn input; MCS output; PSDULen output; rst input
function [MCS,PSDULen] = HTSigBitRecover(bit,validIn,rst)
%#codegen
persistent bitXORVal;
persistent countVal;
persistent mcsBitReg;
persistent psduLenReg;
persistent Pow2Reg;
persistent Pow2Reg1;
persistent psduLenRegDelay;
persistent MCSDelay;


if isempty(bitXORVal)||rst
    bitXORVal = false;
    countVal = uint8(0);
    mcsBitReg = uint16(0); % default for MCS 0
    psduLenReg = fi(0,0,17,0);
    psduLenRegDelay = fi(0,0,17,0);
    Pow2Reg = uint16([1,2,4,8,16,32,64,128,256,512,1024,2048,4096,8192,16384,32768]); % Starts with LSB
    Pow2Reg1 = uint16([1,2,4,8,16,32,64]);
    MCSDelay = uint8(0);
    
end

MCS = uint8(MCSDelay);
PSDULen = fi(psduLenRegDelay,0,17,0);

if validIn
    countVal(:) = countVal + 1;
    if countVal <= 24
        if countVal <= 7
            if bit == 1
                mcsBitReg(:) = mcsBitReg + Pow2Reg1(countVal) ;
            end
        end
        if countVal == 7
            % For SISO MCS is in range [0 7]
            switch(mcsBitReg)
                case 0
                    MCS = uint8(0);
                case 1
                    MCS = uint8(1);
                case 2
                    MCS = uint8(2);
                case 3
                    MCS = uint8(3);
                case 4
                    MCS = uint8(4);
                case 5
                    MCS = uint8(5);
                case 6
                    MCS = uint8(6);
                case 7
                    MCS = uint8(7);
                otherwise
                    MCS = uint8(0);
            end
            MCSDelay = MCS;
        end
        if countVal >= 9
            if bit == 1
                psduLenReg(:) = psduLenReg +  Pow2Reg(countVal-8);
            end
        end
        bitXORVal = bitxor(bitXORVal,bit);
        if countVal == 24
            PSDULen = psduLenReg;
            psduLenRegDelay(:) = psduLenReg;
        else
            PSDULen = fi(psduLenRegDelay,0,17,0);
        end
    
    end

end

end

== matlab function soc_WLAN_fpga/WLAN/WLAN HDL/WLAN_Tx_Rx/WLAN_Rx/WLANHDLReceiver/DataRecovery/Deinterleaver/DeInterleaver_HT/Stage 2 BPSK/Generate Ready/MATLAB Function1 ==
  data: trigger input; out output; nClocks parameter
function out = holdPulse(trigger,nClocks)
%#codegen

 persistent count state;
 if isempty(count)
     count = fi(0,0,nextpow2(nClocks+2),0,hdlfimath);
     state = false;
 end
 
 
 %% Executes in current clock cycle
 if trigger
     state = true;
     count(:) = 0;
 end
 
 if(state && ~trigger)
     count(:) = count +1;
 end
 
 if(count(:) == (nClocks))
    state = false;
 end
     
 out = state;
 
end

== matlab function soc_WLAN_fpga/WLAN/WLAN HDL/WLAN_Tx_Rx/WLAN_Rx/WLANHDLReceiver/DataRecovery/Deinterleaver/DeInterleaver_HT/Stage 2 BPSK/Read Logic/MATLAB Function ==
  data: trigger input; out output; nClocks parameter
function out = holdPulse(trigger,nClocks)
%#codegen

 persistent count state;
 if isempty(count)
     count = fi(0,0,nextpow2(nClocks+1),0,hdlfimath);
     state = false;
 end
 
 %% Executes in next clock cycle
 if(count(:) == (nClocks))
    state = false;
 end
     
 out = state;
 
 
 %% Executes in current clock cycle
 if trigger
     state = true;
     count(:) = 0;
 end
 
 if(state && ~trigger)
     count(:) = count +1;
 end
 
end

== matlab function soc_WLAN_fpga/WLAN/WLAN HDL/WLAN_Tx_Rx/WLAN_Rx/WLANHDLReceiver/WLANTimeAndFrequencySynchronization/Fine CFO Estimation and Correction/Fine CFO Correction/DTConverter ==
  data: dataIn1 input; dataOut output; dataIn2 input
function dataOut = DTConverter(dataIn1,dataIn2)
%#codegen
dataOut = cast(dataIn2,'like',dataIn1);
end

== matlab function soc_WLAN_fpga/WLAN/WLAN HDL/WLAN_Tx_Rx/WLAN_Rx/WLANHDLReceiver/DataRecovery/Deinterleaver/mapmodSelTobps ==
  data: modSel input; bps output
function bps = mapmodSelTobps(modSel)
%#codegen

switch(modSel)
    case 0
        bps = fi(1,0,16,0);
    case 1
        bps = fi(2,0,16,0);
    case 4
        bps = fi(3,0,16,0);
    case 6
        bps = fi(4,0,16,0);
    otherwise
        
        bps = fi(1,0,16,0);
end

== matlab function soc_WLAN_fpga/WLAN/WLAN HDL/WLAN_Tx_Rx/WLAN_Rx/WLANHDLReceiver/DataRecovery/Deinterleaver/DeInterleaver_HT/Stage 2 QPSK/Generate Ready/MATLAB Function1 ==
  data: trigger input; out output; nClocks parameter
function out = holdPulse(trigger,nClocks)
%#codegen

 persistent count state;
 if isempty(count)
     count = fi(0,0,nextpow2(nClocks+2),0,hdlfimath);
     state = false;
 end
 
 
 %% Executes in current clock cycle
 if trigger
     state = true;
     count(:) = 0;
 end
 
 if(state && ~trigger)
     count(:) = count +1;
 end
 
 if(count(:) == (nClocks))
    state = false;
 end
     
 out = state;
 
end

== matlab function soc_WLAN_fpga/WLAN/WLAN HDL/WLAN_Tx_Rx/WLAN_Rx/WLANHDLReceiver/DataRecovery/Deinterleaver/DeInterleaver_HT/Stage 2 QPSK/Read Logic/MATLAB Function ==
  data: trigger input; out output; nClocks parameter
function out = holdPulse(trigger,nClocks)
%#codegen

 persistent count state;
 if isempty(count)
     count = fi(0,0,nextpow2(nClocks+1),0,hdlfimath);
     state = false;
 end
 
 %% Executes in next clock cycle
 if(count(:) == (nClocks))
    state = false;
 end
     
 out = state;
 
 
 %% Executes in current clock cycle
 if trigger
     state = true;
     count(:) = 0;
 end
 
 if(state && ~trigger)
     count(:) = count +1;
 end
 
end

== matlab function soc_WLAN_fpga/WLAN/WLAN HDL/WLAN_Tx_Rx/WLAN_Rx/WLANHDLReceiver/DataRecovery/Deinterleaver/DeInterleaver_HT/Stage 2 16QAM /Generate Ready/MATLAB Function1 ==
  data: trigger input; out output; nClocks parameter
function out = holdPulse(trigger,nClocks)
%#codegen

 persistent count state;
 if isempty(count)
     count = fi(0,0,nextpow2(nClocks+2),0,hdlfimath);
     state = false;
 end
 
 
 %% Executes in current clock cycle
 if trigger
     state = true;
     count(:) = 0;
 end
 
 if(state && ~trigger)
     count(:) = count +1;
 end
 
 if(count(:) == (nClocks))
    state = false;
 end
     
 out = state;
 
end

== matlab function soc_WLAN_fpga/WLAN/WLAN HDL/WLAN_Tx_Rx/WLAN_Rx/WLANHDLReceiver/DataRecovery/Deinterleaver/DeInterleaver_HT/Stage 2 16QAM /Read Logic/MATLAB Function ==
  data: trigger input; out output; nClocks parameter
function out = holdPulse(trigger,nClocks)
%#codegen

 persistent count state;
 if isempty(count)
     count = fi(0,0,nextpow2(nClocks+1),0,hdlfimath);
     state = false;
 end
 
 %% Executes in next clock cycle
 if(count(:) == (nClocks))
    state = false;
 end
     
 out = state;
 
 
 %% Executes in current clock cycle
 if trigger
     state = true;
     count(:) = 0;
 end
 
 if(state && ~trigger)
     count(:) = count +1;
 end
 
end

== matlab function soc_WLAN_fpga/WLAN/WLAN HDL/WLAN_Tx_Rx/WLAN_Rx/WLANHDLReceiver/DataRecovery/Deinterleaver/DeInterleaver_HT/Stage 2 64QAM/Generate Ready/MATLAB Function1 ==
  data: trigger input; out output; nClocks parameter
function out = holdPulse(trigger,nClocks)
%#codegen

 persistent count state;
 if isempty(count)
     count = fi(0,0,nextpow2(nClocks+2),0,hdlfimath);
     state = false;
 end
 
 
 %% Executes in current clock cycle
 if trigger
     state = true;
     count(:) = 0;
 end
 
 if(state && ~trigger)
     count(:) = count +1;
 end
 
 if(count(:) == (nClocks))
    state = false;
 end
     
 out = state;
 
end

== matlab function soc_WLAN_fpga/WLAN/WLAN HDL/WLAN_Tx_Rx/WLAN_Rx/WLANHDLReceiver/DataRecovery/Deinterleaver/DeInterleaver_HT/Stage 2 64QAM/Read Logic/MATLAB Function ==
  data: trigger input; out output; nClocks parameter
function out = holdPulse(trigger,nClocks)
%#codegen

 persistent count state;
 if isempty(count)
     count = fi(0,0,nextpow2(nClocks+1),0,hdlfimath);
     state = false;
 end
 
 %% Executes in next clock cycle
 if(count(:) == (nClocks))
    state = false;
 end
     
 out = state;
 
 
 %% Executes in current clock cycle
 if trigger
     state = true;
     count(:) = 0;
 end
 
 if(state && ~trigger)
     count(:) = count +1;
 end
 
end

== matlab function soc_WLAN_fpga/WLAN/WLAN HDL/WLAN_Tx_Rx/WLAN_Rx/WLANHDLReceiver/DataRecovery/Decoder/Depuncturer/Depuncturer2/puncVecSelector ==
  data: start input; puncVec output; codeRate input
function puncVec = puncVecSlector(start, codeRate)
%#codegen
persistent puncVecDelay;

if isempty(puncVecDelay)
    puncVecDelay =  fi([0 0 0 0 0 0 1 1 1 0].',0,1,0); % default 2/3
end
if start==1
    switch(codeRate)
        case 1 % 2/3
          puncVecDelay = fi([0 0 0 0 0 0 1 1 1 0].',0,1,0);
          
        case 2 % 3/4
          puncVecDelay = fi([0 0 0 0 1 1 1 0 0 1].',0,1,0);
          
        case 3 % 5/6
          puncVecDelay = fi([1 1 1 0 0 1 1 0 0 1].',0,1,0);
        otherwise % default 2/3
          puncVecDelay =  fi([0 0 0 0 0 0 1 1 1 0].',0,1,0);
    end
end
puncVec = puncVecDelay;

== matlab function soc_WLAN_fpga/WLAN/WLAN HDL/WLAN_Tx_Rx/WLAN_Rx/WLANHDLReceiver/DataRecovery/Deinterleaver/DeInterleaver_NonHT/Stage 2 BPSK/Generate Ready/MATLAB Function1 ==
  data: trigger input; out output; nClocks parameter
function out = holdPulse(trigger,nClocks)
%#codegen

 persistent count state;
 if isempty(count)
     count = fi(0,0,nextpow2(nClocks+2),0,hdlfimath);
     state = false;
 end
 
 
 %% Executes in current clock cycle
 if trigger
     state = true;
     count(:) = 0;
 end
 
 if(state && ~trigger)
     count(:) = count +1;
 end
 
 if(count(:) == (nClocks))
    state = false;
 end
     
 out = state;
 
end

== matlab function soc_WLAN_fpga/WLAN/WLAN HDL/WLAN_Tx_Rx/WLAN_Rx/WLANHDLReceiver/DataRecovery/Deinterleaver/DeInterleaver_NonHT/Stage 2 BPSK/Read Logic/MATLAB Function ==
  data: trigger input; out output; nClocks parameter
function out = holdPulse(trigger,nClocks)
%#codegen

 persistent count state;
 if isempty(count)
     count = fi(0,0,nextpow2(nClocks+1),0,hdlfimath);
     state = false;
 end
 
 %% Executes in next clock cycle
 if(count(:) == (nClocks))
    state = false;
 end
     
 out = state;
 
 
 %% Executes in current clock cycle
 if trigger
     state = true;
     count(:) = 0;
 end
 
 if(state && ~trigger)
     count(:) = count +1;
 end
 
end

== matlab function soc_WLAN_fpga/WLAN/WLAN HDL/WLAN_Tx_Rx/WLAN_Rx/WLANHDLReceiver/DataRecovery/Deinterleaver/DeInterleaver_NonHT/Stage 2 QPSK/Generate Ready/MATLAB Function1 ==
  data: trigger input; out output; nClocks parameter
function out = holdPulse(trigger,nClocks)
%#codegen

 persistent count state;
 if isempty(count)
     count = fi(0,0,nextpow2(nClocks+2),0,hdlfimath);
     state = false;
 end
 
 
 %% Executes in current clock cycle
 if trigger
     state = true;
     count(:) = 0;
 end
 
 if(state && ~trigger)
     count(:) = count +1;
 end
 
 if(count(:) == (nClocks))
    state = false;
 end
     
 out = state;
 
end

== matlab function soc_WLAN_fpga/WLAN/WLAN HDL/WLAN_Tx_Rx/WLAN_Rx/WLANHDLReceiver/DataRecovery/Decoder/vhtSigB/vhtSigBDecoding/interpretVHTSigB ==
  data: bit input; psduLen output; validIn input; countVal input; reset input

function psduLen = interpretVHTSigB(bit,validIn,countVal,reset)
%#codegen
persistent Pow2Reg;
persistent psduLenReg;
persistent psduLenRegDelay;

if isempty(Pow2Reg) || reset
    Pow2Reg = fi(2.^(0:16),0,17,0); % Starts with LSB
    psduLenReg = fi(0,0,17,0);
    psduLenRegDelay = fi(0,0,17,0);
end
if countVal <=16 && validIn
    if bit == 1
        psduLenReg(:) = psduLenReg +  Pow2Reg(countVal+1);
    end
end
if countVal == 16
    psduLen = fi(psduLenReg,0,17,0);
    psduLenRegDelay(:) = psduLenReg;
else
    psduLen = fi(psduLenRegDelay,0,17,0);
end

== matlab function soc_WLAN_fpga/WLAN/WLAN HDL/WLAN_Tx_Rx/WLAN_Rx/WLANHDLReceiver/DataRecovery/Deinterleaver/DeInterleaver_NonHT/Stage 2 QPSK/Read Logic/MATLAB Function ==
  data: trigger input; out output; nClocks parameter
function out = holdPulse(trigger,nClocks)
%#codegen

 persistent count state;
 if isempty(count)
     count = fi(0,0,nextpow2(nClocks+1),0,hdlfimath);
     state = false;
 end
 
 %% Executes in next clock cycle
 if(count(:) == (nClocks))
    state = false;
 end
     
 out = state;
 
 
 %% Executes in current clock cycle
 if trigger
     state = true;
     count(:) = 0;
 end
 
 if(state && ~trigger)
     count(:) = count +1;
 end
 
end

== matlab function soc_WLAN_fpga/WLAN/WLAN HDL/WLAN_Tx_Rx/WLAN_Rx/WLANHDLReceiver/FrameFormatDetectionAndSignalRecovery/CRCCheckAndBitInterpretation/VHTSigBitRecover ==
  data: bit input; validIn input; MCS output; rst input; numSTS output
function [MCS,numSTS]  = VHTSigBitRecover(bit,validIn,rst)
%#codegen
persistent bitXORVal;
persistent countVal;
persistent mcsBitReg;

persistent Pow2Reg1;

persistent MCSDelay;
persistent numSTSDelay;
persistent numSTSBitReg;

if isempty(bitXORVal)||rst
    bitXORVal = false;
    countVal = uint8(0);
    mcsBitReg = uint16(0); % default for MCS 0
    Pow2Reg1 = uint16([1,2,4,8]); % 4 bit MCS
    MCSDelay = uint8(0);
    numSTSBitReg = uint16(0);
    numSTSDelay = uint8(0);

end

MCS = uint8(MCSDelay);
numSTS = uint8(numSTSDelay);

if validIn
    countVal(:) = countVal + 1;    
    if countVal <= 25+8
        if countVal <= 24+8 && countVal >= 24+5
            if bit == 1
                mcsBitReg(:) = mcsBitReg + Pow2Reg1(countVal-28) ; %24+4
            end
        end
        if countVal == 24+8
            % For SISO MCS is in range [0 7]
            switch(mcsBitReg)
                case 0 
                    MCS = uint8(0);
                case 1 
                    MCS = uint8(1);
                case 2 
                    MCS = uint8(2);
                case 3 
                    MCS = uint8(3);
                case 4
                    MCS = uint8(4);
                case 5 
                    MCS = uint8(5);
                case 6 
                    MCS = uint8(6);
                case 7 
                    MCS = uint8(7);
                otherwise
                    MCS = uint8(0);
            end
            MCSDelay = MCS;
        end   

        if countVal <= 13 && countVal >= 11
            if bit == 1
                numSTSBitReg(:) = numSTSBitReg + Pow2Reg1(countVal-10) ; %10
            end
        end
        if countVal == 13
            numSTS = uint8(numSTSBitReg+1);
        end
        numSTSDelay = numSTS;
        
    end
end

== matlab function soc_WLAN_fpga/WLAN/WLAN HDL/WLAN_Tx_Rx/WLAN_Rx/WLANHDLReceiver/DataRecovery/symbolDemodulator/sampleAndHold ==
  data: modSelIn input; codeRateIn input; modSelOut output; enb input; reset input; codeRateOut output
function [modSelOut,codeRateOut] = sampleAndHold(modSelIn,codeRateIn,enb,reset)
%#codegen

persistent modSelVal;
persistent codeRateVal;
if isempty(modSelVal) || reset
    modSelVal = fi(0,0,3,0);
    codeRateVal = fi(0,0,2,0);
end

if enb 
    modSelVal(:) = modSelIn;
    codeRateVal(:) = codeRateIn;
end

modSelOut = modSelVal;
codeRateOut = codeRateVal;
